simulink model "ControlLabPracticeDE"  (R2020b)
settings: Solver=VariableStepAuto  StartTime=0.0  StopTime=10.0  RelTol=1e-3
values from neighbouring files (symbols this model uses):
  b = 0.08    [ControlLabPractice.m]
  Bv = 0.003    [ControlLabPractice.m]
  J1 = 0.222    [ControlLabPractice.m]
  J2 = 0.022    [ControlLabPractice.m]
  k = 8    [ControlLabPractice.m]
  Ke = 1.28    [ControlLabPractice.m]
  Kt = 1.25    [ControlLabPractice.m]
  La = 1.21    [ControlLabPractice.m]
  Ra = 11.2    [ControlLabPractice.m]
settings Model: Creator=auamai  LastModifiedBy=auamai

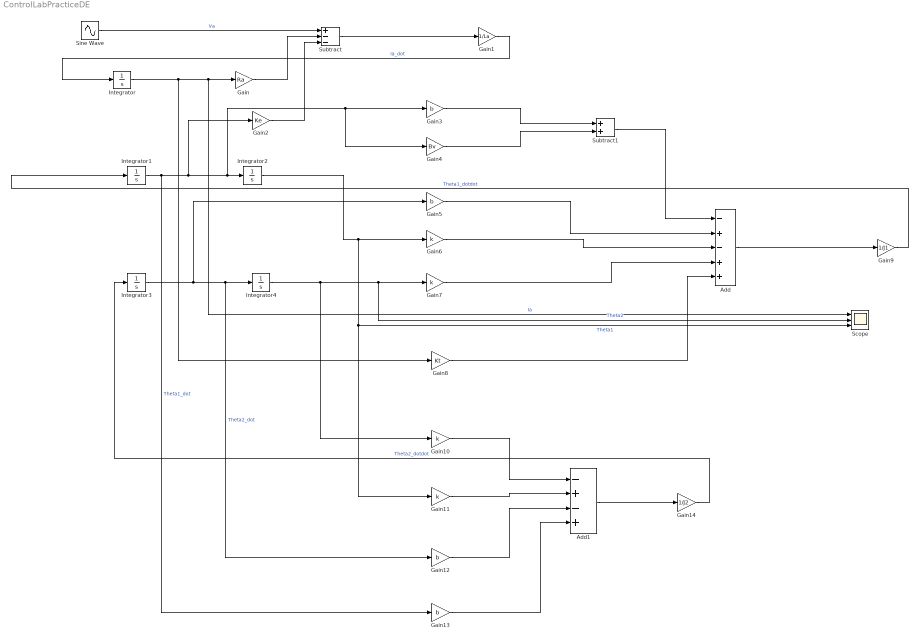
== system ControlLabPracticeDE ==
  Add : Sum  Inputs=-+-++
  Add1 : Sum  Inputs=-+-+
  Gain : Gain  Gain=Ra
  Gain1 : Gain  Gain=1/La
  Gain{6..7,10..11} (4 alike) : Gain  Gain=k
  Gain{3,5,12..13} (4 alike) : Gain  Gain=b
  Gain14 : Gain  Gain=1/J2
  Gain2 : Gain  Gain=Ke
  Gain4 : Gain  Gain=Bv
  Gain8 : Gain  Gain=Kt
  Gain9 : Gain  Gain=1/J1
  Integrator{,1..4} (5 alike) : Integrator
  Scope : Scope  NumInputPorts=3
  Sine Wave : Sin  Frequency=20  SampleTime=0
  Subtract : Sum  Inputs=+--
  Subtract1 : Sum
  wires:
  Gain1/1 -> Integrator/1  "Ia_dot"
  Integrator/1 -> Gain8/1, Scope/1, Gain/1  "Ia"
  Sine Wave/1 -> Subtract/1  "Va"
  Gain/1 -> Subtract/2
  Subtract/1 -> Gain1/1
  Integrator1/1 -> Gain13/1, Gain2/1, Gain4/1, Gain3/1, Integrator2/1  "Theta1_dot"
  Gain9/1 -> Integrator1/1  "Theta1_dotdot"
  Integrator2/1 -> Gain11/1, Scope/3, Gain6/1  "Theta1"
  Gain2/1 -> Subtract/3
  Gain3/1 -> Subtract1/1
  Gain4/1 -> Subtract1/2
  Subtract1/1 -> Add/1
  Integrator3/1 -> Gain5/1, Gain12/1, Integrator4/1  "Theta2_dot"
  Integrator4/1 -> Gain10/1, Scope/2, Gain7/1  "Theta2"
  Gain14/1 -> Integrator3/1  "Theta2_dotdot"
  Gain5/1 -> Add/2
  Gain6/1 -> Add/3
  Gain7/1 -> Add/4
  Gain8/1 -> Add/5
  Add/1 -> Gain9/1
  Gain10/1 -> Add1/1
  Gain11/1 -> Add1/2
  Gain12/1 -> Add1/3
  Gain13/1 -> Add1/4
  Add1/1 -> Gain14/1
